simulink model "Triggered_Subsystem"  (R2021a)
settings: Solver=VariableStepAuto  StartTime=0.0  StopTime=10.0  RelTol=1e-3
settings Model: Creator=lenovo  LastModifiedBy=lenovo

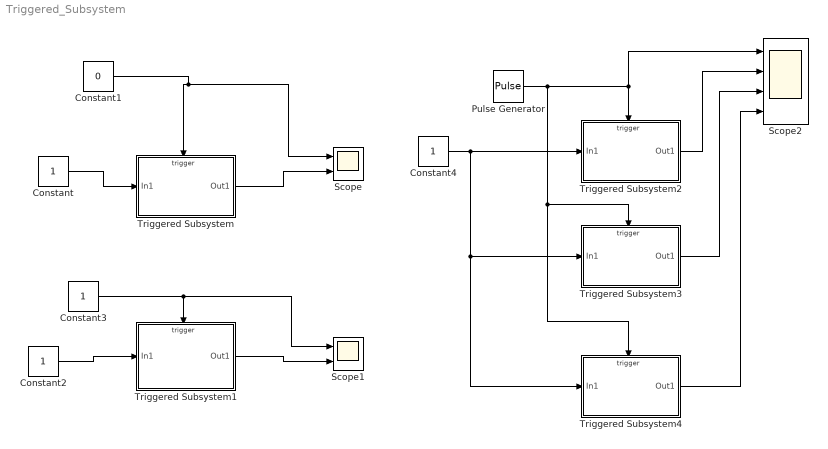
== system Triggered_Subsystem ==
  Constant{,2..4} (4 alike) : Constant
  Constant1 : Constant  Value=0
  Pulse Generator : DiscretePulseGenerator  PulseType=Time based  PulseWidth=50
  Scope : Scope  NumInputPorts=2
  Scope1 : Scope  NumInputPorts=2
  Scope2 : Scope  NumInputPorts=4
  Triggered Subsystem : Subsystem  TreatAsAtomicUnit=on
  Triggered Subsystem1 : Subsystem  TreatAsAtomicUnit=on
  Triggered Subsystem2 : Subsystem  TreatAsAtomicUnit=on
  Triggered Subsystem3 : Subsystem  TreatAsAtomicUnit=on
  Triggered Subsystem4 : Subsystem  TreatAsAtomicUnit=on
  wires:
  Constant/1 -> Triggered Subsystem/1(In1)
  Triggered Subsystem/1(Out1) -> Scope/2
  Constant1/1 -> Scope/1, Triggered Subsystem/Trigger
  Constant2/1 -> Triggered Subsystem1/1(In1)
  Constant3/1 -> Scope1/1, Triggered Subsystem1/Trigger
  Triggered Subsystem1/1(Out1) -> Scope1/2
  Constant4/1 -> Triggered Subsystem2/1(In1), Triggered Subsystem4/1(In1), Triggered Subsystem3/1(In1)
  Pulse Generator/1 -> Triggered Subsystem4/Trigger, Triggered Subsystem3/Trigger, Triggered Subsystem2/Trigger, Scope2/1
  Triggered Subsystem2/1(Out1) -> Scope2/2
  Triggered Subsystem3/1(Out1) -> Scope2/3
  Triggered Subsystem4/1(Out1) -> Scope2/4

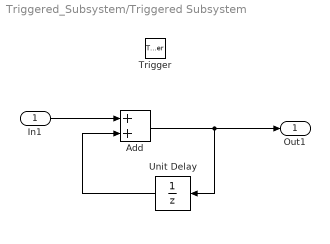
== system Triggered_Subsystem/Triggered Subsystem ==
  In1 : Inport
  Trigger : TriggerPort  VariantControl=(inherit)
  Add : Sum
  Unit Delay : UnitDelay  SampleTime=-1  HasFrameUpgradeWarning=on
  Out1 : Outport
  wires:
  Add/1 -> Out1/1, Unit Delay/1
  In1/1 -> Add/1
  Unit Delay/1 -> Add/2

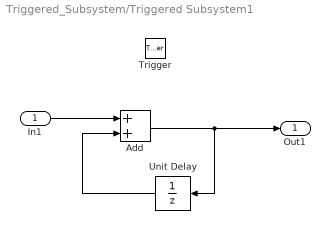
== system Triggered_Subsystem/Triggered Subsystem1 ==
  In1 : Inport
  Trigger : TriggerPort  VariantControl=(inherit)
  Add : Sum
  Unit Delay : UnitDelay  SampleTime=-1  HasFrameUpgradeWarning=on
  Out1 : Outport
  wires:
  Unit Delay/1 -> Add/2
  In1/1 -> Add/1
  Add/1 -> Unit Delay/1, Out1/1

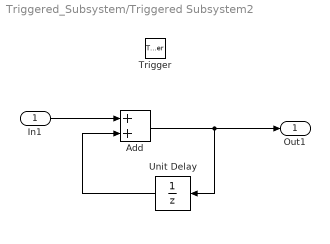
== system Triggered_Subsystem/Triggered Subsystem2 ==
  In1 : Inport
  Trigger : TriggerPort  VariantControl=(inherit)
  Add : Sum
  Unit Delay : UnitDelay  SampleTime=-1  HasFrameUpgradeWarning=on
  Out1 : Outport
  wires:
  Unit Delay/1 -> Add/2
  In1/1 -> Add/1
  Add/1 -> Unit Delay/1, Out1/1

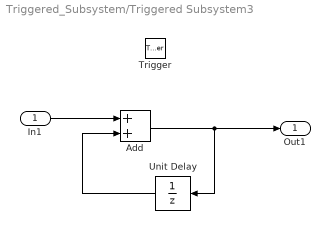
== system Triggered_Subsystem/Triggered Subsystem3 ==
  In1 : Inport
  Trigger : TriggerPort  TriggerType=falling  VariantControl=(inherit)
  Add : Sum
  Unit Delay : UnitDelay  SampleTime=-1  HasFrameUpgradeWarning=on
  Out1 : Outport
  wires:
  Add/1 -> Out1/1, Unit Delay/1
  In1/1 -> Add/1
  Unit Delay/1 -> Add/2

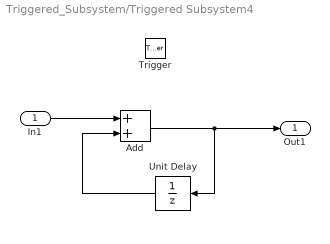
== system Triggered_Subsystem/Triggered Subsystem4 ==
  In1 : Inport
  Trigger : TriggerPort  TriggerType=either  VariantControl=(inherit)
  Add : Sum
  Unit Delay : UnitDelay  SampleTime=-1  HasFrameUpgradeWarning=on
  Out1 : Outport
  wires:
  Unit Delay/1 -> Add/2
  In1/1 -> Add/1
  Add/1 -> Unit Delay/1, Out1/1
